simulink model "GraphFun1_tmp"  (Simulink 8.3)
settings: Solver=FixedStepDiscrete  StartTime=0.0  StopTime=inf  RelTol=1e-3
settings Model: Creator=scaife  LastModifiedBy=hbourbou  CovSFcnEnable=on  ExtModeAutoUpdateStatusClock=off
settings OptimizationCC: InitFltsAndDblsToZero=on
settings DebuggingCC: AlgebraicLoopMsg=error  SaveWithParameterizedLinksMsg=none  SignalResolutionControl=TryResolveAllWithWarning  MultiTaskDSMMsg=warning  MultiTaskCondExecSysMsg=none  FrameProcessingCompatibilityMsg=error  StateNameClashWarn=none
settings SFSimCC: SimParseCustomCode=off
settings GRTTargetCC: TargetFcnLib=ansi_tfl_tmw.mat  GeneratePreprocessorConditionals=Use local settings

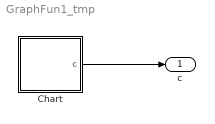
== system GraphFun1_tmp ==
  Chart : Stateflow chart  TreatAsAtomicUnit=on
      settings: PermitHierarchicalResolution=ParametersOnly
  c : Outport
  wires:
  Chart/1(c) -> c/1

== stateflow chart Chart ==
  state A/
    en:a=3;b=4
  state B/
    en:a=5;b=12
  state z=f(x,y) [function]
    (default) -> (junction 9) : {z=sqrt(x*x+y*y);}
  (default) -> A
  A -> B : {c=f(a,b)}
  B -> A : {c=f(a,b)}
  data: x function_input double; y function_input double; z function_output double; a local double; b local double; c output double
